simulink model "Model1"  (R2019b)
settings: Solver=VariableStepAuto  StartTime=0.0  StopTime=time  FixedStep=0.01  RelTol=1e-3
values from neighbouring files (symbols this model uses):
  breath = 60/f    (= 3)    [Model_main.m]
  E1 = 16    [Model_main.m]
  insptime = (ieratio(1)/(ieratio(1)+ieratio(2)))*100    [Model_main.m]
  Pcontrol = 15    [Model_main.m]
  PEEP = 5    [Model_main.m]
  R1 = 15    [Model_main.m]
  V0 = 2    [Model_main.m]
settings Model: Creator=Amne  LastModifiedBy=Amne
settings DataIOCC: ReturnWorkspaceOutputsName=SDOSimTest_Log
settings DebuggingCC: ArithmeticOperatorsInVariantConditions=warning
settings SFSimCC: SimUseLocalCustomCode=off  CustomCodeUndefinedFunction=UseInterfaceOnly
settings RTWCC: RTWUseLocalCustomCode=off

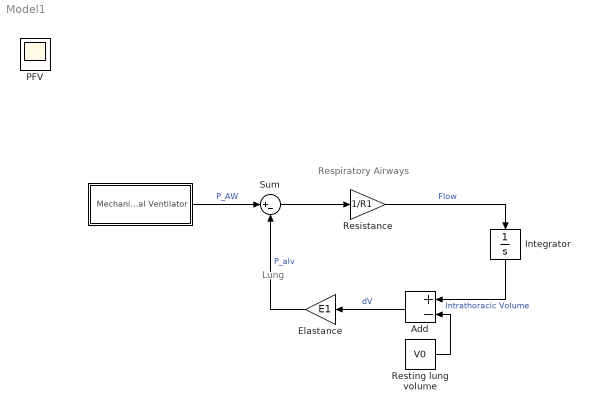
== system Model1 ==
  note: Lung
  note: Respiratory Airways
  " " : Subsystem
  Add : Sum  Inputs=+-
  Elastance : Gain  Gain=E1
  Integrator : Integrator  ZeroCross=off
  Resistance : Gain  Gain=1/R1
  Resting lung volume : Constant  Value=V0
  Sum : Sum  Inputs=|+-
  PFV : Scope
  wires:
  Integrator/1 -> Add/1  "Intrathoracic Volume"
  Elastance/1 -> Sum/2  "P_alv"
  Resistance/1 -> Integrator/1  "Flow"
  Sum/1 -> Resistance/1
  Add/1 -> Elastance/1  "dV"
  Resting lung volume/1 -> Add/2
  " "/1("Mechanical Ventilator ") -> Sum/1  "P_AW"

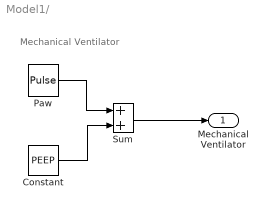
== system Model1/  ==
  note: Mechanical Ventilator
  Constant : Constant  Value=PEEP  SampleTime=0.1
  Paw : DiscretePulseGenerator  PulseType=Time based  Amplitude=Pcontrol  Period=breath  PulseWidth=insptime  PhaseDelay=2  SampleTime=0.1
  Sum : Sum
  "Mechanical Ventilator " : Outport  VectorParamsAs1DForOutWhenUnconnected=off
  wires:
  Paw/1 -> Sum/1
  Constant/1 -> Sum/2
  Sum/1 -> "Mechanical Ventilator "/1
